simulink model "mpu6050_lowpass_filter"  (R2023b)
settings: Solver=FixedStepDiscrete  StartTime=0.0  StopTime=inf  FixedStep=0.01  RelTol=1e-3
undefined symbols (not defined in the file or in its folder): K
libraries: instrumentseriallib x3
settings Model: Creator=mly  LastModifiedBy=mly

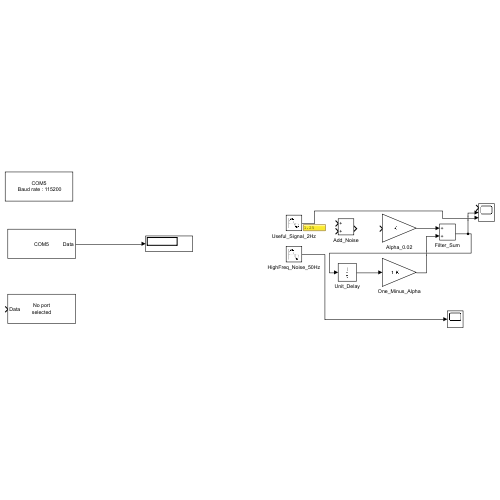
[thumbnail: Simulink's stored preview of the top-level diagram]
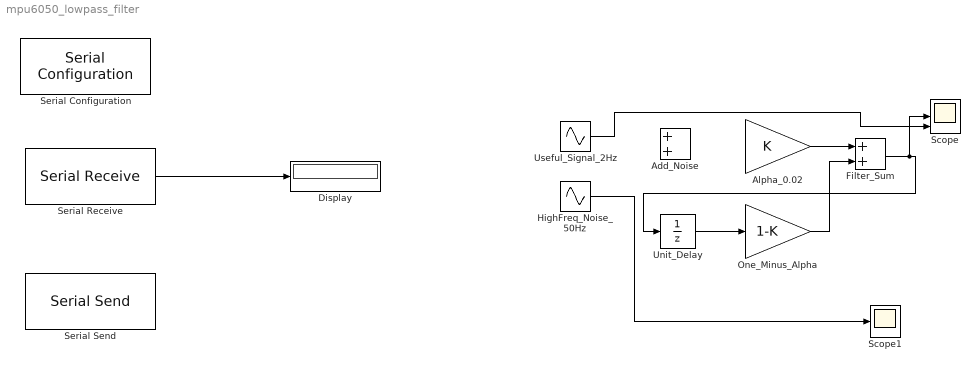
== system mpu6050_lowpass_filter ==
  Add_Noise : Sum
  Alpha_0.02 : Gain  Gain=K
  Display : Display
  Filter_Sum : Sum
  HighFreq_Noise_50Hz : Sin  Amplitude=3  Frequency=2*pi*50  SampleTime=0.005
  One_Minus_Alpha : Gain  Gain=1-K
  Scope : Scope  NumInputPorts=3
  Scope1 : Scope
  Serial Configuration : instrumentseriallib/Serial Configuration  Priority=-200000  PortSel=COM5  Port=COM5  ComPort=COM5  BaudRate=115200  DataBits=8  Parity=none  StopBits=1  ByteOrder=little-endian  FlowControl=none  Timeout=5  SimulateUsing=Interpreted execution  BlockInModel=on  aMode=1
  Serial Receive : instrumentseriallib/Serial Receive  Priority=1  PortSel=COM5  Port=<Select a port...>  ComPort=COM5  DataType=uint8  SaveDataType=uint8  ToggleHeader=off  Header=[]  ToggleTerminator=off  Terminator=<none>  CustomTerminator=[]  InputFormat=Column major  ToggleDataSize=on  DataSize=[1 1]  EnableBlockingMode=on  ActionDataUnavailable=Output last received value  ActionWhenDataUnavailable=Output last received value  CustomValue=0  SampleTime=0.01  SimulateUsing=Interpreted execution  BlockInModel=on  aMode=1
  Serial Send : instrumentseriallib/Serial Send  Priority=1  PortSel=<Select a port...>  Port=<Select a port...>  ComPort=<Select a port...>  Header=[]  Terminator=<none>  CustomTerminator=[]  EnableBlockingMode=on  SimulateUsing=Interpreted execution  BlockInModel=on  aMode=1
  Unit_Delay : UnitDelay  SampleTime=0.01  HasFrameUpgradeWarning=on
  Useful_Signal_2Hz : Sin  Amplitude=10  Frequency=2*pi*2  SampleTime=0.01
  wires:
  One_Minus_Alpha/1 -> Filter_Sum/2
  Useful_Signal_2Hz/1 -> Scope/3
  HighFreq_Noise_50Hz/1 -> Scope1/1
  Unit_Delay/1 -> One_Minus_Alpha/1
  Alpha_0.02/1 -> Filter_Sum/1
  Filter_Sum/1 -> Scope/2, Unit_Delay/1
  Serial Receive/1 -> Display/1
